simulink model "HANcoder_E407_TTA_Controller_v4"  (R2018b)
settings: Solver=FixedStepDiscrete  StartTime=0.0  StopTime=1  FixedStep=0.01  RelTol=1e-3
PreLoadFcn:
  | librarySetup
  | eval([bdroot,'_startup']) %Calling [modelName]_startup.m
values from neighbouring files (symbols this model uses):
  Backup_Board = 0    [HANcoder_E407_TTA_Controller_v3_5_startup.m]    (also in HANcoder_E407_TTA_Controller_v4_6_startup.m; HANcoder_E407_TTA_Controller_v4_7_startup.m; HANcoder_E407_TTA_Controller_v4_startup.m)
  basic_cycle_duration_bc0 = TM_Reset_Board   + COMP_duration    (= 212)    [HANcoder_E407_TTA_Controller_v3_5_startup.m]    (also in HANcoder_E407_TTA_Controller_v4_6_startup.m; HANcoder_E407_TTA_Controller_v4_7_startup.m; HANcoder_E407_TTA_Controller_v4_startup.m)
  basic_cycle_duration_bc1 = TM_Reset_Var_bc1 + COMP_duration    (= 288)    [HANcoder_E407_TTA_Controller_v3_5_startup.m]    (also in HANcoder_E407_TTA_Controller_v4_6_startup.m = 332; HANcoder_E407_TTA_Controller_v4_7_startup.m = 372; HANcoder_E407_TTA_Controller_v4_startup.m = 332)
  comm_delay_estimation1 = round(comm_delay_measured1*hardware_granularity/frequency_IRQ)    [HANcoder_E407_TTA_Controller_v3_5_startup.m]    (also in HANcoder_E407_TTA_Controller_v4_6_startup.m; HANcoder_E407_TTA_Controller_v4_7_startup.m; HANcoder_E407_TTA_Controller_v4_startup.m)
  comm_delay_estimation2 = round(comm_delay_measured2*hardware_granularity/frequency_IRQ)    [HANcoder_E407_TTA_Controller_v3_5_startup.m]    (also in HANcoder_E407_TTA_Controller_v4_6_startup.m; HANcoder_E407_TTA_Controller_v4_7_startup.m; HANcoder_E407_TTA_Controller_v4_startup.m)
  COMM_Period = 40    [HANcoder_E407_TTA_Controller_v3_5_startup.m]    (also in HANcoder_E407_TTA_Controller_v4_6_startup.m; HANcoder_E407_TTA_Controller_v4_7_startup.m; HANcoder_E407_TTA_Controller_v4_startup.m)
  COMM_Phase1 = Simulink.Parameter    [HANcoder_E407_TTA_Controller_v3_5_startup.m]    (also in HANcoder_E407_TTA_Controller_v4_6_startup.m; HANcoder_E407_TTA_Controller_v4_7_startup.m; HANcoder_E407_TTA_Controller_v4_startup.m)
  COMM_Phase2 = Simulink.Parameter    [HANcoder_E407_TTA_Controller_v3_5_startup.m]    (also in HANcoder_E407_TTA_Controller_v4_6_startup.m; HANcoder_E407_TTA_Controller_v4_7_startup.m; HANcoder_E407_TTA_Controller_v4_startup.m)
  COMM_Phase_init1 = Simulink.Parameter    [HANcoder_E407_TTA_Controller_v3_5_startup.m]    (also in HANcoder_E407_TTA_Controller_v4_6_startup.m; HANcoder_E407_TTA_Controller_v4_7_startup.m; HANcoder_E407_TTA_Controller_v4_startup.m)
  COMM_Phase_init2 = Simulink.Parameter    [HANcoder_E407_TTA_Controller_v3_5_startup.m]    (also in HANcoder_E407_TTA_Controller_v4_6_startup.m; HANcoder_E407_TTA_Controller_v4_7_startup.m; HANcoder_E407_TTA_Controller_v4_startup.m)
  COMP_duration = 4    [HANcoder_E407_TTA_Controller_v3_5_startup.m]    (also in HANcoder_E407_TTA_Controller_v4_6_startup.m; HANcoder_E407_TTA_Controller_v4_7_startup.m; HANcoder_E407_TTA_Controller_v4_startup.m)
  Controller1_Board = 1    [HANcoder_E407_TTA_Controller_v3_5_startup.m]    (also in HANcoder_E407_TTA_Controller_v4_6_startup.m; HANcoder_E407_TTA_Controller_v4_7_startup.m; HANcoder_E407_TTA_Controller_v4_startup.m)
  Controller2_Board = 2    [HANcoder_E407_TTA_Controller_v3_5_startup.m]    (also in HANcoder_E407_TTA_Controller_v4_6_startup.m; HANcoder_E407_TTA_Controller_v4_7_startup.m; HANcoder_E407_TTA_Controller_v4_startup.m)
  Controller3_Board = 3    [HANcoder_E407_TTA_Controller_v3_5_startup.m]    (also in HANcoder_E407_TTA_Controller_v4_6_startup.m; HANcoder_E407_TTA_Controller_v4_7_startup.m; HANcoder_E407_TTA_Controller_v4_startup.m)
  delta_a_set = Simulink.Parameter    [HANcoder_E407_TTA_Controller_v3_5_startup.m]    (also in HANcoder_E407_TTA_Controller_v4_6_startup.m; HANcoder_E407_TTA_Controller_v4_7_startup.m; HANcoder_E407_TTA_Controller_v4_startup.m)
  delta_f_set = Simulink.Parameter    [HANcoder_E407_TTA_Controller_v3_5_startup.m]    (also in HANcoder_E407_TTA_Controller_v4_6_startup.m; HANcoder_E407_TTA_Controller_v4_7_startup.m; HANcoder_E407_TTA_Controller_v4_startup.m)
  delta_max = 1    [HANcoder_E407_TTA_Controller_v3_5_startup.m]    (also in HANcoder_E407_TTA_Controller_v4_6_startup.m; HANcoder_E407_TTA_Controller_v4_7_startup.m; HANcoder_E407_TTA_Controller_v4_startup.m)
  delta_min = -1    [HANcoder_E407_TTA_Controller_v3_5_startup.m]    (also in HANcoder_E407_TTA_Controller_v4_6_startup.m; HANcoder_E407_TTA_Controller_v4_7_startup.m; HANcoder_E407_TTA_Controller_v4_startup.m)
  delta_precision = 6    [HANcoder_E407_TTA_Controller_v3_5_startup.m]    (also in HANcoder_E407_TTA_Controller_v4_6_startup.m; HANcoder_E407_TTA_Controller_v4_7_startup.m; HANcoder_E407_TTA_Controller_v4_startup.m)
  e_width = 0.1    [HANcoder_E407_TTA_Controller_v3_5_startup.m]    (also in HANcoder_E407_TTA_Controller_v4_6_startup.m; HANcoder_E407_TTA_Controller_v4_7_startup.m; HANcoder_E407_TTA_Controller_v4_startup.m)
  frequency_IRQ = 100    [HANcoder_E407_2xCAN_TEST_startup.m]    (also in HANcoder_E407_TTA_Controller_v3_5_startup.m; HANcoder_E407_TTA_Controller_v4_6_startup.m; HANcoder_E407_TTA_Controller_v4_7_startup.m; HANcoder_E407_TTA_Controller_v4_startup.m)
  HANtuneOverride = Simulink.Parameter    [HANcoder_E407_2xCAN_TEST_startup.m]    (also in HANcoder_E407_TTA_Controller_v3_5_startup.m; HANcoder_E407_TTA_Controller_v4_6_startup.m; HANcoder_E407_TTA_Controller_v4_7_startup.m; HANcoder_E407_TTA_Controller_v4_startup.m)
  hardware_granularity = 1000000    [HANcoder_E407_2xCAN_TEST_startup.m]    (also in HANcoder_E407_TTA_Controller_v3_5_startup.m; HANcoder_E407_TTA_Controller_v4_6_startup.m; HANcoder_E407_TTA_Controller_v4_7_startup.m; HANcoder_E407_TTA_Controller_v4_startup.m)
  I_a = 2.25    [HANcoder_E407_TTA_Controller_v3_5_startup.m]    (also in HANcoder_E407_TTA_Controller_v4_6_startup.m; HANcoder_E407_TTA_Controller_v4_7_startup.m; HANcoder_E407_TTA_Controller_v4_startup.m)
  I_f = 2.25    [HANcoder_E407_TTA_Controller_v3_5_startup.m]    (also in HANcoder_E407_TTA_Controller_v4_6_startup.m; HANcoder_E407_TTA_Controller_v4_7_startup.m; HANcoder_E407_TTA_Controller_v4_startup.m)
  idle_time_init = basic_cycle_duration_bc0 + basic_cycle_duration_bc1    (= 500)    [HANcoder_E407_TTA_Controller_v3_5_startup.m]    (also in HANcoder_E407_TTA_Controller_v4_6_startup.m = 544; HANcoder_E407_TTA_Controller_v4_7_startup.m = 584; HANcoder_E407_TTA_Controller_v4_startup.m = 544)
  Input_Gen_Board = 4    [HANcoder_E407_TTA_Controller_v3_5_startup.m]    (also in HANcoder_E407_TTA_Controller_v4_6_startup.m; HANcoder_E407_TTA_Controller_v4_7_startup.m; HANcoder_E407_TTA_Controller_v4_startup.m)
  LA_Clock_Gr = 1    [HANcoder_E407_TTA_Controller_v3_5_startup.m]    (also in HANcoder_E407_TTA_Controller_v4_6_startup.m; HANcoder_E407_TTA_Controller_v4_7_startup.m; HANcoder_E407_TTA_Controller_v4_startup.m)
  LA_COMM_dly = 1    [HANcoder_E407_TTA_Controller_v3_5_startup.m]    (also in HANcoder_E407_TTA_Controller_v4_6_startup.m; HANcoder_E407_TTA_Controller_v4_7_startup.m; HANcoder_E407_TTA_Controller_v4_startup.m)
  LA_COMM_Err = 1    [HANcoder_E407_TTA_Controller_v3_5_startup.m]    (also in HANcoder_E407_TTA_Controller_v4_6_startup.m; HANcoder_E407_TTA_Controller_v4_7_startup.m; HANcoder_E407_TTA_Controller_v4_startup.m)
  LA_E_Desync = 1    [HANcoder_E407_TTA_Controller_v3_5_startup.m]    (also in HANcoder_E407_TTA_Controller_v4_6_startup.m; HANcoder_E407_TTA_Controller_v4_7_startup.m; HANcoder_E407_TTA_Controller_v4_startup.m)
  LA_MEX_Flag = 1    [HANcoder_E407_TTA_Controller_v3_5_startup.m]    (also in HANcoder_E407_TTA_Controller_v4_6_startup.m; HANcoder_E407_TTA_Controller_v4_7_startup.m; HANcoder_E407_TTA_Controller_v4_startup.m)
  LA_Task_Act = 1    [HANcoder_E407_TTA_Controller_v3_5_startup.m]    (also in HANcoder_E407_TTA_Controller_v4_6_startup.m; HANcoder_E407_TTA_Controller_v4_7_startup.m; HANcoder_E407_TTA_Controller_v4_startup.m)
  m_v = 100.0    (= 100)    [HANcoder_E407_TTA_Controller_v3_5_startup.m]    (also in HANcoder_E407_TTA_Controller_v4_6_startup.m; HANcoder_E407_TTA_Controller_v4_7_startup.m; HANcoder_E407_TTA_Controller_v4_startup.m)
  Master_Role = 1    [HANcoder_E407_TTA_Controller_v3_5_startup.m]    (also in HANcoder_E407_TTA_Controller_v4_6_startup.m; HANcoder_E407_TTA_Controller_v4_7_startup.m; HANcoder_E407_TTA_Controller_v4_startup.m)
  matrix_cycle_duration = basic_cycle_duration_bc0 + basic_cycle_duration_bc1    (= 500)    [HANcoder_E407_TTA_Controller_v3_5_startup.m]    (also in HANcoder_E407_TTA_Controller_v4_6_startup.m = 544; HANcoder_E407_TTA_Controller_v4_7_startup.m = 584; HANcoder_E407_TTA_Controller_v4_startup.m = 544)
  matrix_rows = 2    [HANcoder_E407_TTA_Controller_v3_5_startup.m]    (also in HANcoder_E407_TTA_Controller_v4_6_startup.m; HANcoder_E407_TTA_Controller_v4_7_startup.m; HANcoder_E407_TTA_Controller_v4_startup.m)
  max_desync = 15    [HANcoder_E407_TTA_Controller_v3_5_startup.m]    (also in HANcoder_E407_TTA_Controller_v4_6_startup.m; HANcoder_E407_TTA_Controller_v4_7_startup.m = 30; HANcoder_E407_TTA_Controller_v4_startup.m)
  max_num_msgs_CAN1 = 2^Tx_bit_number-1    (= 7)    [HANcoder_E407_TTA_Controller_v3_5_startup.m]    (also in HANcoder_E407_TTA_Controller_v4_6_startup.m = 15; HANcoder_E407_TTA_Controller_v4_7_startup.m = 15; HANcoder_E407_TTA_Controller_v4_startup.m)
  max_num_msgs_CAN2 = max_num_msgs_CAN1    (= 7)    [HANcoder_E407_TTA_Controller_v3_5_startup.m]    (also in HANcoder_E407_TTA_Controller_v4_6_startup.m = 15; HANcoder_E407_TTA_Controller_v4_7_startup.m = 15; HANcoder_E407_TTA_Controller_v4_startup.m)
  min_desync = (-1)*max_desync    (= -15)    [HANcoder_E407_TTA_Controller_v3_5_startup.m]    (also in HANcoder_E407_TTA_Controller_v4_6_startup.m; HANcoder_E407_TTA_Controller_v4_7_startup.m = -30; HANcoder_E407_TTA_Controller_v4_startup.m)
  OutControl1_ID = 23    [HANcoder_E407_TTA_Controller_v3_5_startup.m]    (also in HANcoder_E407_TTA_Controller_v4_6_startup.m; HANcoder_E407_TTA_Controller_v4_7_startup.m; HANcoder_E407_TTA_Controller_v4_startup.m)
  OutControl2_ID = 24    [HANcoder_E407_TTA_Controller_v3_5_startup.m]    (also in HANcoder_E407_TTA_Controller_v4_6_startup.m; HANcoder_E407_TTA_Controller_v4_7_startup.m; HANcoder_E407_TTA_Controller_v4_startup.m)
  OutEmulator_ID = 25    [HANcoder_E407_TTA_Controller_v3_5_startup.m]    (also in HANcoder_E407_TTA_Controller_v4_6_startup.m = 26; HANcoder_E407_TTA_Controller_v4_7_startup.m = 26; HANcoder_E407_TTA_Controller_v4_startup.m)
  OutMaster_ID = 25    [HANcoder_E407_TTA_Controller_v4_6_startup.m]    (also in HANcoder_E407_TTA_Controller_v4_7_startup.m; HANcoder_E407_TTA_Controller_v4_startup.m = 26)
  R_al = 0.10    (= 0.1)    [HANcoder_E407_TTA_Controller_v3_5_startup.m]    (also in HANcoder_E407_TTA_Controller_v4_6_startup.m; HANcoder_E407_TTA_Controller_v4_7_startup.m; HANcoder_E407_TTA_Controller_v4_startup.m)
  R_ar = 0.10    (= 0.1)    [HANcoder_E407_TTA_Controller_v3_5_startup.m]    (also in HANcoder_E407_TTA_Controller_v4_6_startup.m; HANcoder_E407_TTA_Controller_v4_7_startup.m; HANcoder_E407_TTA_Controller_v4_startup.m)
  R_fl = 0.10    (= 0.1)    [HANcoder_E407_TTA_Controller_v3_5_startup.m]    (also in HANcoder_E407_TTA_Controller_v4_6_startup.m; HANcoder_E407_TTA_Controller_v4_7_startup.m; HANcoder_E407_TTA_Controller_v4_startup.m)
  R_fr = 0.10    (= 0.1)    [HANcoder_E407_TTA_Controller_v3_5_startup.m]    (also in HANcoder_E407_TTA_Controller_v4_6_startup.m; HANcoder_E407_TTA_Controller_v4_7_startup.m; HANcoder_E407_TTA_Controller_v4_startup.m)
  script_run = Simulink.Parameter    [HANcoder_E407_TTA_Controller_v3_5_startup.m]    (also in HANcoder_E407_TTA_Controller_v4_6_startup.m; HANcoder_E407_TTA_Controller_v4_7_startup.m; HANcoder_E407_TTA_Controller_v4_startup.m)
  SensorValues_ID = 22    [HANcoder_E407_TTA_Controller_v3_5_startup.m]    (also in HANcoder_E407_TTA_Controller_v4_6_startup.m; HANcoder_E407_TTA_Controller_v4_7_startup.m; HANcoder_E407_TTA_Controller_v4_startup.m)
  SetValues_ID = 21    [HANcoder_E407_TTA_Controller_v3_5_startup.m]    (also in HANcoder_E407_TTA_Controller_v4_6_startup.m; HANcoder_E407_TTA_Controller_v4_7_startup.m; HANcoder_E407_TTA_Controller_v4_startup.m)
  Slave_Role = 2    [HANcoder_E407_TTA_Controller_v3_5_startup.m]    (also in HANcoder_E407_TTA_Controller_v4_6_startup.m; HANcoder_E407_TTA_Controller_v4_7_startup.m; HANcoder_E407_TTA_Controller_v4_startup.m)
  speed_k_d = Simulink.Parameter    [HANcoder_E407_TTA_Controller_v3_5_startup.m]    (also in HANcoder_E407_TTA_Controller_v4_6_startup.m; HANcoder_E407_TTA_Controller_v4_7_startup.m; HANcoder_E407_TTA_Controller_v4_startup.m)
  speed_k_i = Simulink.Parameter    [HANcoder_E407_TTA_Controller_v3_5_startup.m]    (also in HANcoder_E407_TTA_Controller_v4_6_startup.m; HANcoder_E407_TTA_Controller_v4_7_startup.m; HANcoder_E407_TTA_Controller_v4_startup.m)
  speed_k_p = Simulink.Parameter    [HANcoder_E407_TTA_Controller_v3_5_startup.m]    (also in HANcoder_E407_TTA_Controller_v4_6_startup.m; HANcoder_E407_TTA_Controller_v4_7_startup.m; HANcoder_E407_TTA_Controller_v4_startup.m)
  speed_max = 10    [HANcoder_E407_TTA_Controller_v3_5_startup.m]    (also in HANcoder_E407_TTA_Controller_v4_6_startup.m; HANcoder_E407_TTA_Controller_v4_7_startup.m; HANcoder_E407_TTA_Controller_v4_startup.m)
  speed_min = -10    [HANcoder_E407_TTA_Controller_v3_5_startup.m]    (also in HANcoder_E407_TTA_Controller_v4_6_startup.m; HANcoder_E407_TTA_Controller_v4_7_startup.m; HANcoder_E407_TTA_Controller_v4_startup.m)
  speed_precision = 3    [HANcoder_E407_TTA_Controller_v3_5_startup.m]    (also in HANcoder_E407_TTA_Controller_v4_6_startup.m; HANcoder_E407_TTA_Controller_v4_7_startup.m; HANcoder_E407_TTA_Controller_v4_startup.m)
  Sync_ID = 1    [HANcoder_E407_TTA_Controller_v3_5_startup.m]    (also in HANcoder_E407_TTA_Controller_v4_6_startup.m; HANcoder_E407_TTA_Controller_v4_7_startup.m; HANcoder_E407_TTA_Controller_v4_startup.m)
  tau_max = 5    [HANcoder_E407_TTA_Controller_v3_5_startup.m]    (also in HANcoder_E407_TTA_Controller_v4_6_startup.m; HANcoder_E407_TTA_Controller_v4_7_startup.m; HANcoder_E407_TTA_Controller_v4_startup.m)
  tau_min = -5    [HANcoder_E407_TTA_Controller_v3_5_startup.m]    (also in HANcoder_E407_TTA_Controller_v4_6_startup.m; HANcoder_E407_TTA_Controller_v4_7_startup.m; HANcoder_E407_TTA_Controller_v4_startup.m)
  tau_range = abs(tau_max) + abs(tau_min)    [HANcoder_E407_TTA_Controller_v3_5_startup.m]    (also in HANcoder_E407_TTA_Controller_v4_6_startup.m; HANcoder_E407_TTA_Controller_v4_7_startup.m; HANcoder_E407_TTA_Controller_v4_startup.m)
  theta_max = (speed_max/R_fr)*matrix_cycle_duration*frequency_IRQ/hardware_granularity    (= 5)    [HANcoder_E407_TTA_Controller_v3_5_startup.m]    (also in HANcoder_E407_TTA_Controller_v4_6_startup.m = 5.44; HANcoder_E407_TTA_Controller_v4_7_startup.m = 5.84; HANcoder_E407_TTA_Controller_v4_startup.m = 5.44)
  theta_min = (-1)*theta_max    (= -5)    [HANcoder_E407_TTA_Controller_v3_5_startup.m]    (also in HANcoder_E407_TTA_Controller_v4_6_startup.m = -5.44; HANcoder_E407_TTA_Controller_v4_7_startup.m = -5.84; HANcoder_E407_TTA_Controller_v4_startup.m = -5.44)
  theta_precision = 7-(fix(log2(theta_max))+1)    [HANcoder_E407_TTA_Controller_v3_5_startup.m]    (also in HANcoder_E407_TTA_Controller_v4_6_startup.m; HANcoder_E407_TTA_Controller_v4_7_startup.m; HANcoder_E407_TTA_Controller_v4_startup.m)
  Tl_a = 0.6    [HANcoder_E407_TTA_Controller_v3_5_startup.m]    (also in HANcoder_E407_TTA_Controller_v4_6_startup.m; HANcoder_E407_TTA_Controller_v4_7_startup.m; HANcoder_E407_TTA_Controller_v4_startup.m)
  Tl_f = 0.6    [HANcoder_E407_TTA_Controller_v3_5_startup.m]    (also in HANcoder_E407_TTA_Controller_v4_6_startup.m; HANcoder_E407_TTA_Controller_v4_7_startup.m; HANcoder_E407_TTA_Controller_v4_startup.m)
  TM_Check_Output_Control1 = TM_COMM_Output_Control1 + COMM_duration    (= 188)    [HANcoder_E407_TTA_Controller_v3_5_startup.m]    (also in HANcoder_E407_TTA_Controller_v4_6_startup.m; HANcoder_E407_TTA_Controller_v4_7_startup.m; HANcoder_E407_TTA_Controller_v4_startup.m)
  TM_Check_Output_Control2 = TM_COMM_Output_Control2 + COMM_duration    (= 232)    [HANcoder_E407_TTA_Controller_v3_5_startup.m]    (also in HANcoder_E407_TTA_Controller_v4_6_startup.m; HANcoder_E407_TTA_Controller_v4_7_startup.m; HANcoder_E407_TTA_Controller_v4_startup.m)
  TM_Check_Output_Emulator = TM_COMM_Output_Emulator + COMM_duration    (= 280)    [HANcoder_E407_TTA_Controller_v3_5_startup.m]    (also in HANcoder_E407_TTA_Controller_v4_6_startup.m = 320; HANcoder_E407_TTA_Controller_v4_7_startup.m = 360; HANcoder_E407_TTA_Controller_v4_startup.m = 320)
  TM_Check_Output_Emulator_2 = TM_Check_Output_Emulator + 2    (= 282)    [HANcoder_E407_TTA_Controller_v3_5_startup.m]    (also in HANcoder_E407_TTA_Controller_v4_6_startup.m = 322; HANcoder_E407_TTA_Controller_v4_7_startup.m = 362; HANcoder_E407_TTA_Controller_v4_startup.m = 322)
  TM_Check_Output_Emulator_3 = TM_Check_Output_Emulator_2 + 2    (= 324)    [HANcoder_E407_TTA_Controller_v4_6_startup.m]    (also in HANcoder_E407_TTA_Controller_v4_7_startup.m = 364; HANcoder_E407_TTA_Controller_v4_startup.m)
  TM_Check_Sensor_Values = TM_COMM_Sensor_Values + COMM_duration    (= 132)    [HANcoder_E407_TTA_Controller_v3_5_startup.m]    (also in HANcoder_E407_TTA_Controller_v4_6_startup.m; HANcoder_E407_TTA_Controller_v4_7_startup.m; HANcoder_E407_TTA_Controller_v4_startup.m)
  TM_Check_Sensor_Values_2 = TM_Check_Sensor_Values + 2    (= 134)    [HANcoder_E407_TTA_Controller_v3_5_startup.m]    (also in HANcoder_E407_TTA_Controller_v4_6_startup.m; HANcoder_E407_TTA_Controller_v4_7_startup.m; HANcoder_E407_TTA_Controller_v4_startup.m)
  TM_Check_Set_Values = TM_COMM_Set_Values + COMM_duration    (= 88)    [HANcoder_E407_TTA_Controller_v3_5_startup.m]    (also in HANcoder_E407_TTA_Controller_v4_6_startup.m; HANcoder_E407_TTA_Controller_v4_7_startup.m; HANcoder_E407_TTA_Controller_v4_startup.m)
  TM_Check_Set_Values_2 = TM_Check_Set_Values + 2    (= 90)    [HANcoder_E407_TTA_Controller_v3_5_startup.m]    (also in HANcoder_E407_TTA_Controller_v4_6_startup.m; HANcoder_E407_TTA_Controller_v4_7_startup.m; HANcoder_E407_TTA_Controller_v4_startup.m)
  TM_Check_Sync = TM_COMM_Sync   + COMM_duration    (= 40)    [HANcoder_E407_TTA_Controller_v3_5_startup.m]    (also in HANcoder_E407_TTA_Controller_v4_6_startup.m; HANcoder_E407_TTA_Controller_v4_7_startup.m; HANcoder_E407_TTA_Controller_v4_startup.m)
  TM_Check_TOuts = TM_Count_Vote3 + COMP_duration    (= 196)    [HANcoder_E407_TTA_Controller_v3_5_startup.m]    (also in HANcoder_E407_TTA_Controller_v4_6_startup.m; HANcoder_E407_TTA_Controller_v4_7_startup.m; HANcoder_E407_TTA_Controller_v4_startup.m)
  TM_Check_Vote1 = TM_COMM_Vote1  + COMM_duration    (= 92)    [HANcoder_E407_TTA_Controller_v3_5_startup.m]    (also in HANcoder_E407_TTA_Controller_v4_6_startup.m; HANcoder_E407_TTA_Controller_v4_7_startup.m; HANcoder_E407_TTA_Controller_v4_startup.m)
  TM_Check_Vote2 = TM_COMM_Vote2  + COMM_duration    (= 140)    [HANcoder_E407_TTA_Controller_v3_5_startup.m]    (also in HANcoder_E407_TTA_Controller_v4_6_startup.m; HANcoder_E407_TTA_Controller_v4_7_startup.m; HANcoder_E407_TTA_Controller_v4_startup.m)
  TM_Check_Vote2_2 = TM_Check_Vote2 + 2    (= 142)    [HANcoder_E407_TTA_Controller_v3_5_startup.m]    (also in HANcoder_E407_TTA_Controller_v4_6_startup.m; HANcoder_E407_TTA_Controller_v4_7_startup.m; HANcoder_E407_TTA_Controller_v4_startup.m)
  TM_Check_Vote3 = TM_COMM_Vote3  + COMM_duration    (= 188)    [HANcoder_E407_TTA_Controller_v3_5_startup.m]    (also in HANcoder_E407_TTA_Controller_v4_6_startup.m; HANcoder_E407_TTA_Controller_v4_7_startup.m; HANcoder_E407_TTA_Controller_v4_startup.m)
  TM_COMM_Output_Control1 = TM_Velocity + COMP_duration    (= 148)    [HANcoder_E407_TTA_Controller_v3_5_startup.m]    (also in HANcoder_E407_TTA_Controller_v4_6_startup.m; HANcoder_E407_TTA_Controller_v4_7_startup.m; HANcoder_E407_TTA_Controller_v4_startup.m)
  TM_COMM_Output_Control2 = TM_Check_Output_Control1 + COMP_duration    (= 192)    [HANcoder_E407_TTA_Controller_v3_5_startup.m]    (also in HANcoder_E407_TTA_Controller_v4_6_startup.m; HANcoder_E407_TTA_Controller_v4_7_startup.m; HANcoder_E407_TTA_Controller_v4_startup.m)
  TM_COMM_Output_Emulator = TM_TMR + COMP_duration    (= 240)    [HANcoder_E407_TTA_Controller_v3_5_startup.m]    (also in HANcoder_E407_TTA_Controller_v4_6_startup.m = 280; HANcoder_E407_TTA_Controller_v4_7_startup.m = 320; HANcoder_E407_TTA_Controller_v4_startup.m = 280)
  TM_COMM_Output_Master = TM_Check_Output_Control2 + COMM_duration    (= 272)    [HANcoder_E407_TTA_Controller_v4_6_startup.m]    (also in HANcoder_E407_TTA_Controller_v4_7_startup.m; HANcoder_E407_TTA_Controller_v4_startup.m)
  TM_COMM_Sensor_Values = TM_Check_Set_Values + COMP_duration    (= 92)    [HANcoder_E407_TTA_Controller_v3_5_startup.m]    (also in HANcoder_E407_TTA_Controller_v4_6_startup.m; HANcoder_E407_TTA_Controller_v4_7_startup.m; HANcoder_E407_TTA_Controller_v4_startup.m)
  TM_COMM_Set_Values = TM_Update_LT + COMP_duration    (= 48)    [HANcoder_E407_TTA_Controller_v3_5_startup.m]    (also in HANcoder_E407_TTA_Controller_v4_6_startup.m; HANcoder_E407_TTA_Controller_v4_7_startup.m; HANcoder_E407_TTA_Controller_v4_startup.m)
  TM_COMM_Sync = basic_cycle_start    (= 0)    [HANcoder_E407_TTA_Controller_v3_5_startup.m]    (also in HANcoder_E407_TTA_Controller_v4_6_startup.m; HANcoder_E407_TTA_Controller_v4_7_startup.m; HANcoder_E407_TTA_Controller_v4_startup.m)
  TM_COMM_Vote1 = TM_Vote_Dec    + COMP_duration    (= 52)    [HANcoder_E407_TTA_Controller_v3_5_startup.m]    (also in HANcoder_E407_TTA_Controller_v4_6_startup.m; HANcoder_E407_TTA_Controller_v4_7_startup.m; HANcoder_E407_TTA_Controller_v4_startup.m)
  TM_COMM_Vote2 = TM_Count_Vote1 + COMP_duration    (= 100)    [HANcoder_E407_TTA_Controller_v3_5_startup.m]    (also in HANcoder_E407_TTA_Controller_v4_6_startup.m; HANcoder_E407_TTA_Controller_v4_7_startup.m; HANcoder_E407_TTA_Controller_v4_startup.m)
  TM_COMM_Vote3 = TM_Count_Vote2 + COMP_duration    (= 148)    [HANcoder_E407_TTA_Controller_v3_5_startup.m]    (also in HANcoder_E407_TTA_Controller_v4_6_startup.m; HANcoder_E407_TTA_Controller_v4_7_startup.m; HANcoder_E407_TTA_Controller_v4_startup.m)
  TM_Count_Vote1 = TM_Check_Vote1 + COMP_duration    (= 96)    [HANcoder_E407_TTA_Controller_v3_5_startup.m]    (also in HANcoder_E407_TTA_Controller_v4_6_startup.m; HANcoder_E407_TTA_Controller_v4_7_startup.m; HANcoder_E407_TTA_Controller_v4_startup.m)
  TM_Count_Vote2 = TM_Check_Vote2 + COMP_duration    (= 144)    [HANcoder_E407_TTA_Controller_v3_5_startup.m]    (also in HANcoder_E407_TTA_Controller_v4_6_startup.m; HANcoder_E407_TTA_Controller_v4_7_startup.m; HANcoder_E407_TTA_Controller_v4_startup.m)
  TM_Count_Vote3 = TM_Check_Vote3 + COMP_duration    (= 192)    [HANcoder_E407_TTA_Controller_v3_5_startup.m]    (also in HANcoder_E407_TTA_Controller_v4_6_startup.m; HANcoder_E407_TTA_Controller_v4_7_startup.m; HANcoder_E407_TTA_Controller_v4_startup.m)
  TM_Data_bc0 = TM_COMM_Sync    (= 0)    [HANcoder_E407_TTA_Controller_v3_5_startup.m]    (also in HANcoder_E407_TTA_Controller_v4_6_startup.m; HANcoder_E407_TTA_Controller_v4_7_startup.m; HANcoder_E407_TTA_Controller_v4_startup.m)
  TM_Data_bc1 = TM_Data_bc0(1:4)    [HANcoder_E407_TTA_Controller_v3_5_startup.m]    (also in HANcoder_E407_TTA_Controller_v4_6_startup.m; HANcoder_E407_TTA_Controller_v4_7_startup.m; HANcoder_E407_TTA_Controller_v4_startup.m)
  TM_New_Master = TM_Check_TOuts + COMP_duration    (= 200)    [HANcoder_E407_TTA_Controller_v3_5_startup.m]    (also in HANcoder_E407_TTA_Controller_v4_6_startup.m; HANcoder_E407_TTA_Controller_v4_7_startup.m; HANcoder_E407_TTA_Controller_v4_startup.m)
  TM_Reset_Board = TM_Reset_Var   + COMP_duration    (= 208)    [HANcoder_E407_TTA_Controller_v3_5_startup.m]    (also in HANcoder_E407_TTA_Controller_v4_6_startup.m; HANcoder_E407_TTA_Controller_v4_7_startup.m; HANcoder_E407_TTA_Controller_v4_startup.m)
  TM_Reset_Var = TM_New_Master  + COMP_duration    (= 204)    [HANcoder_E407_TTA_Controller_v3_5_startup.m]    (also in HANcoder_E407_TTA_Controller_v4_6_startup.m; HANcoder_E407_TTA_Controller_v4_7_startup.m; HANcoder_E407_TTA_Controller_v4_startup.m)
  TM_Reset_Var_bc1 = TM_Check_Output_Emulator + COMP_duration    (= 284)    [HANcoder_E407_TTA_Controller_v3_5_startup.m]    (also in HANcoder_E407_TTA_Controller_v4_6_startup.m = 328; HANcoder_E407_TTA_Controller_v4_7_startup.m = 368; HANcoder_E407_TTA_Controller_v4_startup.m = 328)
  TM_Reset_Var_bc1_2 = TM_Reset_Var_bc1 + 2    (= 286)    [HANcoder_E407_TTA_Controller_v3_5_startup.m]    (also in HANcoder_E407_TTA_Controller_v4_6_startup.m = 330; HANcoder_E407_TTA_Controller_v4_7_startup.m = 370; HANcoder_E407_TTA_Controller_v4_startup.m = 330)
  TM_Steer = TM_Check_Sensor_Values + COMP_duration    (= 136)    [HANcoder_E407_TTA_Controller_v3_5_startup.m]    (also in HANcoder_E407_TTA_Controller_v4_6_startup.m; HANcoder_E407_TTA_Controller_v4_7_startup.m; HANcoder_E407_TTA_Controller_v4_startup.m)
  TM_TMR = TM_Check_Output_Control2 + COMP_duration    (= 236)    [HANcoder_E407_TTA_Controller_v3_5_startup.m]    (also in HANcoder_E407_TTA_Controller_v4_6_startup.m = 276; HANcoder_E407_TTA_Controller_v4_7_startup.m = 316; HANcoder_E407_TTA_Controller_v4_startup.m = 276)
  TM_TMR_2 = TM_TMR + 1    (= 237)    [HANcoder_E407_TTA_Controller_v3_5_startup.m]    (also in HANcoder_E407_TTA_Controller_v4_6_startup.m = 277; HANcoder_E407_TTA_Controller_v4_7_startup.m = 317; HANcoder_E407_TTA_Controller_v4_startup.m = 277)
  TM_TMR_3 = TM_TMR + 3    (= 239)    [HANcoder_E407_TTA_Controller_v3_5_startup.m]    (also in HANcoder_E407_TTA_Controller_v4_6_startup.m = 279; HANcoder_E407_TTA_Controller_v4_7_startup.m = 319; HANcoder_E407_TTA_Controller_v4_startup.m = 279)
  TM_Torque = TM_Steer + COMP_duration    (= 140)    [HANcoder_E407_TTA_Controller_v3_5_startup.m]    (also in HANcoder_E407_TTA_Controller_v4_6_startup.m; HANcoder_E407_TTA_Controller_v4_7_startup.m; HANcoder_E407_TTA_Controller_v4_startup.m)
  TM_Type_bc0 = COMM    (= 0)    [HANcoder_E407_TTA_Controller_v3_5_startup.m]    (also in HANcoder_E407_TTA_Controller_v4_6_startup.m; HANcoder_E407_TTA_Controller_v4_7_startup.m; HANcoder_E407_TTA_Controller_v4_startup.m)
  TM_Type_bc1 = TM_Type_bc0(1:4)    [HANcoder_E407_TTA_Controller_v3_5_startup.m]    (also in HANcoder_E407_TTA_Controller_v4_6_startup.m; HANcoder_E407_TTA_Controller_v4_7_startup.m; HANcoder_E407_TTA_Controller_v4_startup.m)
  TM_Update_LT = TM_Check_Sync  + COMP_duration    (= 44)    [HANcoder_E407_TTA_Controller_v3_5_startup.m]    (also in HANcoder_E407_TTA_Controller_v4_6_startup.m; HANcoder_E407_TTA_Controller_v4_7_startup.m; HANcoder_E407_TTA_Controller_v4_startup.m)
  TM_Update_LT_2 = TM_Update_LT   + 2    (= 46)    [HANcoder_E407_TTA_Controller_v3_5_startup.m]    (also in HANcoder_E407_TTA_Controller_v4_6_startup.m; HANcoder_E407_TTA_Controller_v4_7_startup.m; HANcoder_E407_TTA_Controller_v4_startup.m)
  TM_Velocity = TM_Torque + COMP_duration    (= 144)    [HANcoder_E407_TTA_Controller_v3_5_startup.m]    (also in HANcoder_E407_TTA_Controller_v4_6_startup.m; HANcoder_E407_TTA_Controller_v4_7_startup.m; HANcoder_E407_TTA_Controller_v4_startup.m)
  TM_Vote_Dec = TM_Update_LT   + COMP_duration    (= 48)    [HANcoder_E407_TTA_Controller_v3_5_startup.m]    (also in HANcoder_E407_TTA_Controller_v4_6_startup.m; HANcoder_E407_TTA_Controller_v4_7_startup.m; HANcoder_E407_TTA_Controller_v4_startup.m)
  TM_Vote_Dec_2 = TM_Vote_Dec    + 2    (= 50)    [HANcoder_E407_TTA_Controller_v3_5_startup.m]    (also in HANcoder_E407_TTA_Controller_v4_6_startup.m; HANcoder_E407_TTA_Controller_v4_7_startup.m; HANcoder_E407_TTA_Controller_v4_startup.m)
  torque_a_k_d = Simulink.Parameter    [HANcoder_E407_TTA_Controller_v3_5_startup.m]    (also in HANcoder_E407_TTA_Controller_v4_6_startup.m; HANcoder_E407_TTA_Controller_v4_7_startup.m; HANcoder_E407_TTA_Controller_v4_startup.m)
  torque_a_k_i = Simulink.Parameter    [HANcoder_E407_TTA_Controller_v3_5_startup.m]    (also in HANcoder_E407_TTA_Controller_v4_6_startup.m; HANcoder_E407_TTA_Controller_v4_7_startup.m; HANcoder_E407_TTA_Controller_v4_startup.m)
  torque_a_k_p = Simulink.Parameter    [HANcoder_E407_TTA_Controller_v3_5_startup.m]    (also in HANcoder_E407_TTA_Controller_v4_6_startup.m; HANcoder_E407_TTA_Controller_v4_7_startup.m; HANcoder_E407_TTA_Controller_v4_startup.m)
  torque_f_k_d = Simulink.Parameter    [HANcoder_E407_TTA_Controller_v3_5_startup.m]    (also in HANcoder_E407_TTA_Controller_v4_6_startup.m; HANcoder_E407_TTA_Controller_v4_7_startup.m; HANcoder_E407_TTA_Controller_v4_startup.m)
  torque_f_k_i = Simulink.Parameter    [HANcoder_E407_TTA_Controller_v3_5_startup.m]    (also in HANcoder_E407_TTA_Controller_v4_6_startup.m; HANcoder_E407_TTA_Controller_v4_7_startup.m; HANcoder_E407_TTA_Controller_v4_startup.m)
  ... (+7 more)
undefined symbols (not defined in the file or in its folder): A0, A1, A2, A3, A4, CON2, CON3, CON4, D10, D12, D13, D2, D3, D8, D9
libraries: hdlsllib x452, HANcoder_STM32_Target x30, simulink x3, simulink_extras x1
(part 2 of 79)

== system HANcoder_E407_TTA_Controller_v4/HANcoder STM32 Target - E407-STM32 algorithm/TTA CAN System/CAN1 Recieve ==
  note: Function call counter
  Trigger : TriggerPort  TriggerType=function-call  VariantControl=Variant  PortDimensions=1
  AND2 : Logic  IconShape=distinctive  AllPortsSameDT=off  OutDataTypeStr=boolean
  AND3 : Logic  IconShape=distinctive  AllPortsSameDT=off  OutDataTypeStr=boolean
  Buffer ready : Subsystem  TreatAsAtomicUnit=on
  Constant : Constant  Value=0
  Constant3 : Constant  OutDataTypeStr=uint32
  Constant4 : Constant
  Constant5 : Constant  Value=2
  Constant6 : Constant  Value=0
  Constant7 : Constant
  Data Store Memory1 : DataStoreMemory  DataStoreName=fcn_call_counter  ReadBeforeWriteMsg=warning  WriteAfterWriteMsg=warning  WriteAfterReadMsg=warning  ShowAdditionalParam=off  OutDataTypeStr=uint32
  Data Store Read : DataStoreRead  DataStoreName=RxID_CAN1
  Data Store Read1 : DataStoreRead  DataStoreName=fcn_call_counter
  Data Store Read10 : DataStoreRead  DataStoreName=Rx_State_CAN1
  Data Store Read4 : DataStoreRead  DataStoreName=Rx_State_CAN1
  Data Store Read9 : DataStoreRead  DataStoreName=Rx_State_CAN1
  Data Store Write : DataStoreWrite  DataStoreName=fcn_call_counter
  Equal{3,5..7} (4 alike) : RelationalOperator  Operator===  OutDataTypeStr=boolean  RndMeth=Simplest
  Equal4 : RelationalOperator  OutDataTypeStr=boolean  RndMeth=Simplest
  Prepare buffer : Subsystem  TreatAsAtomicUnit=on
  RxID_CAN : Subsystem
  Sum1 : Sum
  Update message buffers : Subsystem
  wires:
  AND3/1 -> Update message buffers/Enable
  Data Store Read/1 -> RxID_CAN/1(RxID)  "RxID_CAN1_s"
  RxID_CAN/2(message) -> Update message buffers/1(message)
  Constant7/1 -> Equal6/2
  Constant6/1 -> Equal5/2
  RxID_CAN/1(CAN_new) -> Equal4/1, Equal3/2
  Constant5/1 -> Equal7/2
  Equal5/1 -> Prepare buffer/Enable
  Data Store Read9/1 -> Equal7/1
  Equal4/1 -> AND3/2
  Equal6/1 -> AND2/1
  Equal3/1 -> AND2/2
  AND2/1 -> Buffer ready/Enable
  Equal7/1 -> AND3/1
  Data Store Read10/1 -> Equal6/1
  Constant/1 -> Equal3/1
  Data Store Read4/1 -> Equal5/1
  Data Store Read1/1 -> Sum1/2
  Constant3/1 -> Sum1/1
  Sum1/1 -> Data Store Write/1  "RxCAN1_counter_s"
  Constant4/1 -> Equal4/2

== system HANcoder_E407_TTA_Controller_v4/HANcoder STM32 Target - E407-STM32 algorithm/TTA CAN System/CAN1 Send ==
  note: Logic Analyzer - COMM Delay
  note: Logic Analyzer - DEBUG
  note: DEBUG
  note: Function call counter
  note: Logic Analyzer - DEBUG
      | Message in transmission!
  note: Transmission message count
      | Update
  Trigger : TriggerPort  TriggerType=function-call  VariantControl=Variant  PortDimensions=1
  AND : Logic  IconShape=distinctive  AllPortsSameDT=off  OutDataTypeStr=boolean
  Bus Selector : BusSelector  OutputSignals=Buffer_1,Buffer_2,Buffer_3,Buffer_4,Buffer_5,Buffer_6,Buffer_7,Buffer_8
  CAN send : Subsystem  Tag=HANcoder_TARGET_STM32_E407  AncestorBlock=HANcoder_STM32_Target/STM32-E407/CAN/CAN/CAN send  mask(CAN send){canBus=CAN 1, frameType=Standard (11 bit), inputNumber=8, dataType=uint8, byteOrder=off, tsamp=-1}
      mask prompts: canBus "CAN channel"; frameType "Identifier type"; inputNumber "Input ports"; dataType "Input datatype"; byteOrder "Byte order: Checked = MSB first, unchecked = LSB first."; tsamp "Sample time"
      mask help:
      | Function
      | ==========
      | Send a message on the CAN channel.
      |
      | Parameters
      | ==========
      | CAN channel:           The CAN channel to send the message on.
      | Identifier type:         normal or extended ID's
      | Input ports:              The amount of input ports
      | Input datatype:        The datatype of the input ports
      | Byte order:               Select MSB or LSB first
      | Sample time:            -1 or divisible by base sample time [seconds]
      |
      | Input
      | ==========
      | Port 1:                   CAN ID(uint32) in hexadecimal ie: hex2dec('0a')
      | Port 2..9                CAN message data
      mask init:
      | sfcn_can_send_mcb(canBus, frameType, inputNumber, dataType, byteOrder)
      settings: MoveFcn=drawLogos
      mask Help: web('sfcn_can_send.html');
      mask TypeOptions canBus: CAN 1 | CAN 2
      mask TypeOptions frameType: Standard (11 bit) | Extended (29 bit)
      mask TypeOptions dataType: int8 | uint8 | int16 | uint16 | int32 | uint32 | boolean
      mask Display:
      | fprintf('Send on\nCAN %x', canBus);
      | port_label('input', 1, 'ID');patch([135 141 141],[8 14 2],[1 0 0]);patch([143 143 149],[14 2 8],[0 0 0.35]);
  Cast To Double : DataTypeConversion  OutDataTypeStr=double
  Constant : Constant  OutDataTypeStr=boolean
  Constant1 : Constant  Value=Sync_ID
  Constant2 : Constant  Value=LA_COMM_dly
  Constant3 : Constant  OutDataTypeStr=uint32
  Constant8 : Constant  Priority=2
  Data Store Memory1 : DataStoreMemory  DataStoreName=fcn_call_counter  ReadBeforeWriteMsg=warning  WriteAfterWriteMsg=warning  WriteAfterReadMsg=warning  ShowAdditionalParam=off  OutDataTypeStr=uint32
  Data Store Read : DataStoreRead  DataStoreName=fcn_call_counter
  Data Store Read1 : DataStoreRead  DataStoreName=TxID_CAN1
  Data Store Read2 : DataStoreRead  DataStoreName=Msg_Tx_CAN1
  Data Store Read3 : DataStoreRead  DataStoreName=TxID_CAN1
  Data Store Read4 : DataStoreRead  Priority=1  DataStoreName=Tx_msg_count_CAN1
  Data Store Write : DataStoreWrite  DataStoreName=fcn_call_counter
  Data Store Write1 : DataStoreWrite  DataStoreName=Toggle_Pin_A0
  Data Store Write2 : DataStoreWrite  Priority=4  DataStoreName=Tx_msg_count_CAN1
  Data Type Conversion{,4..10} (8 alike) : DataTypeConversion  OutDataTypeStr=uint8
  Data Type Conversion1 : DataTypeConversion  OutDataTypeStr=uint32
  Equal : RelationalOperator  Operator===  OutDataTypeStr=boolean  RndMeth=Simplest
  Logic Analyzer - COMM delay measurement : Subsystem  TreatAsAtomicUnit=on
  Plus : Sum  Priority=3
  Sum1 : Sum
  Terminator : Terminator
  wires:
  Data Type Conversion10/1 -> CAN send/9(In9)
  Data Type Conversion/1 -> CAN send/2(In2)
  Data Type Conversion1/1 -> CAN send/1(In1)
  Data Type Conversion9/1 -> CAN send/8(In8)
  Data Type Conversion8/1 -> CAN send/7(In7)
  Data Type Conversion5/1 -> CAN send/4(In4)
  Data Type Conversion4/1 -> CAN send/3(In3)
  Data Type Conversion6/1 -> CAN send/5(In5)
  Data Type Conversion7/1 -> CAN send/6(In6)
  Constant3/1 -> Sum1/1
  Data Store Read/1 -> Sum1/2
  Sum1/1 -> Data Store Write/1  "TxCAN1_counter_s"
  Constant/1 -> Data Store Write1/1
  Data Store Read2/1 -> Bus Selector/1
  Bus Selector/2 -> Data Type Conversion4/1  "<Buffer_2>"
  Bus Selector/3 -> Data Type Conversion5/1  "<Buffer_3>"
  Bus Selector/4 -> Data Type Conversion6/1  "<Buffer_4>"
  Bus Selector/5 -> Data Type Conversion7/1  "<Buffer_5>"
  Bus Selector/6 -> Data Type Conversion8/1  "<Buffer_6>"
  Bus Selector/7 -> Data Type Conversion9/1  "<Buffer_7>"
  Bus Selector/8 -> Data Type Conversion10/1  "<Buffer_8>"
  Data Store Read3/1 -> Data Type Conversion1/1  "TxID_CAN1_s"
  Constant8/1 -> Plus/2
  Plus/1 -> Data Store Write2/1
  Data Store Read4/1 -> Plus/1
  Cast To Double/1 -> Terminator/1  "Tx_temporal_msg_CAN1"
  Bus Selector/1 -> Cast To Double/1, Data Type Conversion/1  "<Buffer_1>"
  Data Store Read1/1 -> Equal/1
  Constant1/1 -> Equal/2
  Constant2/1 -> AND/2
  AND/1 -> Logic Analyzer - COMM delay measurement/Enable
  Equal/1 -> AND/1

== system HANcoder_E407_TTA_Controller_v4/HANcoder STM32 Target - E407-STM32 algorithm/TTA CAN System/CAN2 Recieve ==
  note: Function call counter
  Trigger : TriggerPort  TriggerType=function-call  VariantControl=Variant  PortDimensions=1
  AND2 : Logic  IconShape=distinctive  AllPortsSameDT=off  OutDataTypeStr=boolean
  AND3 : Logic  IconShape=distinctive  AllPortsSameDT=off  OutDataTypeStr=boolean
  Buffer ready : Subsystem  TreatAsAtomicUnit=on
  Constant : Constant  Value=0
  Constant3 : Constant  OutDataTypeStr=uint32
  Constant4 : Constant
  Constant5 : Constant  Value=2
  Constant6 : Constant  Value=0
  Constant7 : Constant
  Data Store Memory1 : DataStoreMemory  DataStoreName=fcn_call_counter  ReadBeforeWriteMsg=warning  WriteAfterWriteMsg=warning  WriteAfterReadMsg=warning  ShowAdditionalParam=off  OutDataTypeStr=uint32
  Data Store Read : DataStoreRead  DataStoreName=RxID_CAN2
  Data Store Read1 : DataStoreRead  DataStoreName=fcn_call_counter
  Data Store Read10 : DataStoreRead  DataStoreName=Rx_State_CAN2
  Data Store Read4 : DataStoreRead  DataStoreName=Rx_State_CAN2
  Data Store Read9 : DataStoreRead  DataStoreName=Rx_State_CAN2
  Data Store Write : DataStoreWrite  DataStoreName=fcn_call_counter
  Equal{3,5..7} (4 alike) : RelationalOperator  Operator===  OutDataTypeStr=boolean  RndMeth=Simplest
  Equal4 : RelationalOperator  OutDataTypeStr=boolean  RndMeth=Simplest
  Prepare buffer : Subsystem  TreatAsAtomicUnit=on
  RxID_CAN : Subsystem
  Sum1 : Sum
  Update message buffers : Subsystem
  wires:
  Data Store Read4/1 -> Equal5/1
  Constant/1 -> Equal3/1
  Data Store Read10/1 -> Equal6/1
  Equal7/1 -> AND3/1
  AND2/1 -> Buffer ready/Enable
  Equal3/1 -> AND2/2
  Equal6/1 -> AND2/1
  Equal4/1 -> AND3/2
  Data Store Read9/1 -> Equal7/1
  Equal5/1 -> Prepare buffer/Enable
  Constant5/1 -> Equal7/2
  RxID_CAN/1(CAN_new) -> Equal4/1, Equal3/2
  Constant6/1 -> Equal5/2
  Constant7/1 -> Equal6/2
  RxID_CAN/2(message) -> Update message buffers/1(message)
  AND3/1 -> Update message buffers/Enable
  Data Store Read/1 -> RxID_CAN/1(RxID)  "RxID_CAN2_s"
  Sum1/1 -> Data Store Write/1  "RxCAN2_counter_s"
  Data Store Read1/1 -> Sum1/2
  Constant3/1 -> Sum1/1
  Constant4/1 -> Equal4/2

== system HANcoder_E407_TTA_Controller_v4/HANcoder STM32 Target - E407-STM32 algorithm/TTA CAN System/CAN2 Send ==
  note: Logic Analyzer - DEBUG
      | Message in transmission!
  note: Function call counter
  note: DEBUG
  note: Logic Analyzer - DEBUG
  note: Transmission message count
      | Update
  note: Logic Analyzer - COMM Delay
  Trigger : TriggerPort  TriggerType=function-call  VariantControl=Variant  PortDimensions=1
  AND : Logic  IconShape=distinctive  AllPortsSameDT=off  OutDataTypeStr=boolean
  Bus Selector : BusSelector  OutputSignals=Buffer_1,Buffer_2,Buffer_3,Buffer_4,Buffer_5,Buffer_6,Buffer_7,Buffer_8
  CAN send1 : Subsystem  Tag=HANcoder_TARGET_STM32_E407  AncestorBlock=HANcoder_STM32_Target/STM32-E407/CAN/CAN/CAN send  mask(CAN send){canBus=CAN 2, frameType=Standard (11 bit), inputNumber=8, dataType=uint8, byteOrder=off, tsamp=-1}
      mask prompts: canBus "CAN channel"; frameType "Identifier type"; inputNumber "Input ports"; dataType "Input datatype"; byteOrder "Byte order: Checked = MSB first, unchecked = LSB first."; tsamp "Sample time"
      mask help:
      | Function
      | ==========
      | Send a message on the CAN channel.
      |
      | Parameters
      | ==========
      | CAN channel:           The CAN channel to send the message on.
      | Identifier type:         normal or extended ID's
      | Input ports:              The amount of input ports
      | Input datatype:        The datatype of the input ports
      | Byte order:               Select MSB or LSB first
      | Sample time:            -1 or divisible by base sample time [seconds]
      |
      | Input
      | ==========
      | Port 1:                   CAN ID(uint32) in hexadecimal ie: hex2dec('0a')
      | Port 2..9                CAN message data
      mask init:
      | sfcn_can_send_mcb(canBus, frameType, inputNumber, dataType, byteOrder)
      settings: MoveFcn=drawLogos
      mask Help: web('sfcn_can_send.html');
      mask TypeOptions canBus: CAN 1 | CAN 2
      mask TypeOptions frameType: Standard (11 bit) | Extended (29 bit)
      mask TypeOptions dataType: int8 | uint8 | int16 | uint16 | int32 | uint32 | boolean
      mask Display:
      | fprintf('Send on\nCAN %x', canBus);
      | port_label('input', 1, 'ID');patch([140 146 146],[8 14 2],[1 0 0]);patch([148 148 154],[14 2 8],[0 0 0.35]);
  Cast To Double : DataTypeConversion  OutDataTypeStr=double
  Constant : Constant  OutDataTypeStr=boolean
  Constant1 : Constant  Value=Sync_ID
  Constant2 : Constant  Value=LA_COMM_dly
  Constant3 : Constant  OutDataTypeStr=uint32
  Constant8 : Constant  Priority=2
  Data Store Memory1 : DataStoreMemory  DataStoreName=fcn_call_counter  ReadBeforeWriteMsg=warning  WriteAfterWriteMsg=warning  WriteAfterReadMsg=warning  ShowAdditionalParam=off  OutDataTypeStr=uint32
  Data Store Read : DataStoreRead  DataStoreName=fcn_call_counter
  Data Store Read1 : DataStoreRead  DataStoreName=TxID_CAN2
  Data Store Read2 : DataStoreRead  DataStoreName=Msg_Tx_CAN2
  Data Store Read3 : DataStoreRead  DataStoreName=TxID_CAN2
  Data Store Read4 : DataStoreRead  Priority=1  DataStoreName=Tx_msg_count_CAN2
  Data Store Write : DataStoreWrite  DataStoreName=fcn_call_counter
  Data Store Write1 : DataStoreWrite  DataStoreName=Toggle_Pin_A0
  Data Store Write2 : DataStoreWrite  Priority=4  DataStoreName=Tx_msg_count_CAN2
  Data Type Conversion{,4..10} (8 alike) : DataTypeConversion  OutDataTypeStr=uint8
  Data Type Conversion1 : DataTypeConversion  OutDataTypeStr=uint32
  Equal : RelationalOperator  Operator===  OutDataTypeStr=boolean  RndMeth=Simplest
  Logic Analyzer - COMM delay measurement : Subsystem  TreatAsAtomicUnit=on
  Plus : Sum  Priority=3
  Sum1 : Sum
  Terminator : Terminator
  wires:
  Constant/1 -> Data Store Write1/1
  Sum1/1 -> Data Store Write/1  "TxCAN2_counter_s"
  Data Store Read/1 -> Sum1/2
  Constant3/1 -> Sum1/1
  Data Type Conversion7/1 -> CAN send1/6(In6)
  Data Type Conversion6/1 -> CAN send1/5(In5)
  Data Type Conversion4/1 -> CAN send1/3(In3)
  Data Type Conversion5/1 -> CAN send1/4(In4)
  Data Type Conversion8/1 -> CAN send1/7(In7)
  Data Type Conversion9/1 -> CAN send1/8(In8)
  Data Type Conversion1/1 -> CAN send1/1(In1)
  Data Type Conversion/1 -> CAN send1/2(In2)
  Data Type Conversion10/1 -> CAN send1/9(In9)
  Data Store Read3/1 -> Data Type Conversion1/1  "TxID_CAN2_s"
  Bus Selector/3 -> Data Type Conversion5/1  "<Buffer_3>"
  Bus Selector/2 -> Data Type Conversion4/1  "<Buffer_2>"
  Bus Selector/6 -> Data Type Conversion8/1  "<Buffer_6>"
  Bus Selector/4 -> Data Type Conversion6/1  "<Buffer_4>"
  Bus Selector/8 -> Data Type Conversion10/1  "<Buffer_8>"
  Data Store Read2/1 -> Bus Selector/1
  Bus Selector/7 -> Data Type Conversion9/1  "<Buffer_7>"
  Bus Selector/5 -> Data Type Conversion7/1  "<Buffer_5>"
  Data Store Read4/1 -> Plus/1
  Plus/1 -> Data Store Write2/1
  Constant8/1 -> Plus/2
  Bus Selector/1 -> Cast To Double/1, Data Type Conversion/1  "<Buffer_1>"
  Cast To Double/1 -> Terminator/1  "Tx_temporal_msg_CAN2"
  Constant1/1 -> Equal/2
  Constant2/1 -> AND/2
  AND/1 -> Logic Analyzer - COMM delay measurement/Enable
  Equal/1 -> AND/1
  Data Store Read1/1 -> Equal/1

== system HANcoder_E407_TTA_Controller_v4/HANcoder STM32 Target - E407-STM32 algorithm/TTA CAN System/If Action Subsystem ==
  note: CAN ID Init
  Action Port : ActionPort  ActionType=then
  Add : Sum  Inputs=++++
  Constant : Constant
  Constant1 : Constant  Value=2
  Constant2 : Constant  Value=4
  Constant3 : Constant  Value=8
  Digital Input4 : HANcoder_STM32_Target/STM32-E407/Digital Inputs/Digital Input  Tag=HANcoder_TARGET_STM32_E407  pinID=CON3 - D2 - 5V Tolerant  config=Pulldown  tsamp=-1
      settings: SourceProductName=HANcoder STM32 Target
  Digital Input5 : HANcoder_STM32_Target/STM32-E407/Digital Inputs/Digital Input  Tag=HANcoder_TARGET_STM32_E407  pinID=CON3 - D3 - 5V Tolerant  config=Pulldown  tsamp=-1
      settings: SourceProductName=HANcoder STM32 Target
  Digital Input6 : HANcoder_STM32_Target/STM32-E407/Digital Inputs/Digital Input  Tag=HANcoder_TARGET_STM32_E407  pinID=CON3 - D4 - 5V Tolerant  config=Pulldown  tsamp=-1
      settings: SourceProductName=HANcoder STM32 Target
  Digital Input7 : HANcoder_STM32_Target/STM32-E407/Digital Inputs/Digital Input  Tag=HANcoder_TARGET_STM32_E407  pinID=CON3 - D5 - 5V Tolerant  config=Pulldown  tsamp=-1
      settings: SourceProductName=HANcoder STM32 Target
  Multiply{,1..3} (4 alike) : Product
  Out1 : Outport
  wires:
  Constant1/1 -> Multiply1/1
  Add/1 -> Out1/1
  Constant3/1 -> Multiply3/1
  Constant2/1 -> Multiply2/1
  Multiply2/1 -> Add/3
  Digital Input7/1 -> Multiply3/2
  Digital Input5/1 -> Multiply1/2
  Multiply3/1 -> Add/4
  Multiply1/1 -> Add/2
  Digital Input6/1 -> Multiply2/2
  Multiply/1 -> Add/1
  Digital Input4/1 -> Multiply/2
  Constant/1 -> Multiply/1

== system HANcoder_E407_TTA_Controller_v4/HANcoder STM32 Target - E407-STM32 algorithm/TTA CAN System/If Action Subsystem1 ==
  New_Board_ID : Inport
  Action Port : ActionPort  ActionType=then
  Constant : Constant  OutDataTypeStr=boolean
  Constant1 : Constant  Value=0  OutDataTypeStr=boolean
  Constant2 : Constant  OutDataTypeStr=boolean
  Constant3 : Constant  Value=0  OutDataTypeStr=boolean
  Constant4 : Constant  Value=Controller1_Board
  Constant5 : Constant  Value=Controller2_Board
  Constant6 : Constant  Value=Controller3_Board
  Digital Output : HANcoder_STM32_Target/STM32-E407/Digital Outputs/Digital Output  Tag=HANcoder_TARGET_STM32_E407  pinID=CON3 - D2  config=Push pull  tsamp=-1
      settings: SourceProductName=HANcoder STM32 Target
  Digital Output1 : HANcoder_STM32_Target/STM32-E407/Digital Outputs/Digital Output  Tag=HANcoder_TARGET_STM32_E407  pinID=CON3 - D3  config=Push pull  tsamp=-1
      settings: SourceProductName=HANcoder STM32 Target
  Equal : RelationalOperator  Operator===  OutDataTypeStr=boolean  RndMeth=Simplest
  Equal1 : RelationalOperator  Operator===  OutDataTypeStr=boolean  RndMeth=Simplest
  Equal2 : RelationalOperator  Operator===  OutDataTypeStr=boolean  RndMeth=Simplest
  OR : Logic  Operator=OR  IconShape=distinctive  AllPortsSameDT=off  OutDataTypeStr=boolean
  OR1 : Logic  Operator=OR  IconShape=distinctive  AllPortsSameDT=off  OutDataTypeStr=boolean
  Switch : Switch  Criteria=u2 > Threshold
  Switch1 : Switch  Criteria=u2 > Threshold
  wires:
  Switch/1 -> Digital Output/1
  Switch1/1 -> Digital Output1/1
  Constant2/1 -> Switch/1
  Constant3/1 -> Switch/3
  Constant/1 -> Switch1/1
  Constant1/1 -> Switch1/3
  Equal2/1 -> OR1/1
  Constant4/1 -> Equal/1
  Constant5/1 -> Equal2/1
  Constant6/1 -> Equal1/1
  Equal/1 -> OR/1
  OR/1 -> Switch/2
  Equal1/1 -> OR/2, OR1/2
  OR1/1 -> Switch1/2
  New_Board_ID/1 -> Equal1/2, Equal/2, Equal2/2

== system HANcoder_E407_TTA_Controller_v4/HANcoder STM32 Target - E407-STM32 algorithm/TTA CAN System/Initialize Clock Schedule ==
  Enable : EnablePort
  Constant : Constant  OutDataTypeStr=uint16
  Constant1 : Constant  Value=3  OutDataTypeStr=uint8
  Constant2 : Constant
  Data Store Write : DataStoreWrite  DataStoreName=init_clock
  Schedule Compare Event : HANcoder_STM32_Target/STM32-E407/Timer Outputs/Schedule Compare Event  Tag=HANcoder_TARGET_STM32_E407  pin=TIM4 - CON PD - 15 - 5V Tolerant  tsamp=-1
      settings: SourceProductName=HANcoder STM32 Target
  wires:
  Constant/1 -> Schedule Compare Event/1
  Constant1/1 -> Schedule Compare Event/2
  Constant2/1 -> Data Store Write/1

== system HANcoder_E407_TTA_Controller_v4/HANcoder STM32 Target - E407-STM32 algorithm/TTA CAN System/Local Time generation ==
  note: Reschedule IRQ activation
  Clock_State : Inport
  function : TriggerPort  TriggerType=function-call  VariantControl=Variant
  Chart : Stateflow chart  TreatAsAtomicUnit=on
  Constant : Constant  Value=frequency_IRQ  OutDataTypeStr=uint16
  Constant1 : Constant  Value=3  OutDataTypeStr=uint8
  Constant2 : Constant  OutDataTypeStr=uint16
  Data Store Read : DataStoreRead  DataStoreName=Local_Ticks
  Data Store Read1 : DataStoreRead  DataStoreName=Local_Ticks
  Data Store Write : DataStoreWrite  DataStoreName=Local_Ticks
  Get Last Event Counter : HANcoder_STM32_Target/STM32-E407/Timer Outputs/Get Last Event Counter  Tag=HANcoder_TARGET_STM32_E407  pin=TIM4 - CON PD - 15 - 5V Tolerant  tsamp=-1
      settings: SourceProductName=HANcoder STM32 Target
  Schedule Compare Event1 : HANcoder_STM32_Target/STM32-E407/Timer Outputs/Schedule Compare Event  Tag=HANcoder_TARGET_STM32_E407  pin=TIM4 - CON PD - 15 - 5V Tolerant  tsamp=-1
      settings: SourceProductName=HANcoder STM32 Target
  Sum : Sum
  Sum1 : Sum
  Switch : Switch  Criteria=u2 > Threshold
  activate_CAN_management : Outport
  wires:
  Get Last Event Counter/1 -> Sum/1
  Constant/1 -> Sum/2
  Sum/1 -> Schedule Compare Event1/1
  Constant1/1 -> Schedule Compare Event1/2
  Data Store Read1/1 -> Switch/3
  Data Store Read/1 -> Sum1/1
  Constant2/1 -> Sum1/2
  Clock_State/1 -> Chart/1(Condition), Switch/2
  Switch/1 -> Data Store Write/1  "local_ticks_interrupt"
  Sum1/1 -> Switch/1
  Chart/1(Trigger_Signal()) -> activate_CAN_management/1
